simulink model "torqueBalancingR2015a"  (Simulink 8.5)
settings: Solver=FixedStepDiscrete  StartTime=0.0  StopTime="CONFIG.SIMULATION_TIME "  FixedStep=CONFIG.Ts  RelTol=1e-3
InitFcn:
  | cd(fileparts(which(bdroot)));
  | initTorqueBalancing;
values from neighbouring files (symbols this model uses):
  WBT_robotName = 'iCub'    [initTorqueBalancing.m]
undefined symbols (not defined in the file or in its folder): bVectorConstraints, CONFIG, ConstraintsMatrix, DiscIntNeverNeededParam, gain, references, reg, ROBOT_DOF, ROBOT_DOF_FOR_SIMULINK, sat, SM, sm
libraries: WBToolboxLibrary x141, simulink x6
(part 3 of 4)

== system torqueBalancingR2015a/State Machine/State machine Yoga and Coordinator/State Machine Yoga/visualise inertial/w_H_root_link1 ==
  qj : Inport
  inertial : Inport  Port=2
  "CoM6D ->  CoMXYZ1" : Selector  NumberOfDimensions=2  InputPortWidth=7  IndexOptions=Index vector (dialog),Index vector (dialog)  Indices=[1 2 3],[1 2 3]  OutputSizes=1,1
  Constant2 : Constant  Value=eye(4)
  Constant5 : Constant  Value=eye(4)
  Constant6 : Constant  Value=eye(4)
  Inv\* : Product  Inputs=/*  Multiplication=Matrix(*)
  Inv\*1 : Product  Inputs=/*  Multiplication=Matrix(*)
  Inv\*2 : Product  Inputs=/  Multiplication=Matrix(*)
  Product : Product  Multiplication=Matrix(*)
  Selector : Selector  InputPortWidth=12  IndexOptions=Index vector (dialog)  Indices=[4 5 6 ]  OutputSizes=1
  Subsystem : Subsystem
  Switch6 : Switch  Criteria=u2 > Threshold
  USE_IMU4EST_BASE : Constant  Value=CONFIG.USE_IMU4EST_BASE
  fromImuToHomogeousTransformFCN : MATLAB Function  TreatAsAtomicUnit=on
      settings: PermitHierarchicalResolution=ParametersOnly
  holder 1 : WBToolboxLibrary/Utilities/holder 
  holder 2 : WBToolboxLibrary/Utilities/holder 
  imu : WBToolboxLibrary/wholeBodyModel/Kinematics/Forward Kinematics  frameName='imu_frame'  robotName=WBT_robotName  localName=WBT_modelName  wbiFile=WBT_wbiFilename  wbiList=WBT_wbiList
  l_sole_acc : Scope
      settings: TimeRange=auto  LimitDataPoints=on  MaxDataPoints=5000  SaveToWorkspace=off  SaveName=ScopeData  YMin=-10  YMax=10  SampleTime=-1  DataFormat=Array
  link : WBToolboxLibrary/wholeBodyModel/Kinematics/Forward Kinematics  frameName=link_name  robotName=WBT_robotName  localName=WBT_modelName  wbiFile=WBT_wbiFilename  wbiList=WBT_wbiList
  root_link : WBToolboxLibrary/wholeBodyModel/Kinematics/Forward Kinematics  frameName='root_link'  robotName=WBT_robotName  localName=WBT_modelName  wbiFile=WBT_wbiFilename  wbiList=WBT_wbiList
  w_H_root : Outport
  wires:
  Constant5/1 -> imu/1
  Inv\*/1 -> holder 1/1, fromImuToHomogeousTransformFCN/1(imu_H_link), Inv\*2/1  "imu_H_link"
  imu/1 -> Inv\*/1
  Constant6/1 -> link/1
  Inv\*1/1 -> Switch6/3, fromImuToHomogeousTransformFCN/3(link_H_root)  "link_H_root"
  link/1 -> Inv\*1/1, Inv\*/2
  inertial/1 -> Selector/1, holder 2/1, fromImuToHomogeousTransformFCN/5(inertial)
  Switch6/1 -> w_H_root/1
  USE_IMU4EST_BASE/1 -> Switch6/2
  fromImuToHomogeousTransformFCN/1(w_H_root) -> Switch6/1
  Constant2/1 -> root_link/1
  qj/1 -> root_link/2, link/2, imu/2
  root_link/1 -> Inv\*1/2
  holder 1/1 -> fromImuToHomogeousTransformFCN/2(imu_H_link_0)
  holder 2/1 -> fromImuToHomogeousTransformFCN/4(inertial_0)
  Inv\*2/1 -> "CoM6D ->  CoMXYZ1"/1
  "CoM6D ->  CoMXYZ1"/1 -> Product/1  "l_sole_R_imu"
  Selector/1 -> Product/2  "imu_acce"
  Product/1 -> l_sole_acc/1
  Subsystem/1(Neck Position) -> fromImuToHomogeousTransformFCN/6(neck)

== system torqueBalancingR2015a/State Machine/State machine Yoga and Coordinator/State Machine Yoga/visualise inertial/w_H_root_link2 ==
  qj : Inport
  inertial : Inport  Port=2
  "CoM6D ->  CoMXYZ1" : Selector  NumberOfDimensions=2  InputPortWidth=7  IndexOptions=Index vector (dialog),Index vector (dialog)  Indices=[1 2 3],[1 2 3]  OutputSizes=1,1
  Constant2 : Constant  Value=eye(4)
  Constant5 : Constant  Value=eye(4)
  Constant6 : Constant  Value=eye(4)
  Inv\* : Product  Inputs=/*  Multiplication=Matrix(*)
  Inv\*1 : Product  Inputs=/*  Multiplication=Matrix(*)
  Inv\*2 : Product  Inputs=/  Multiplication=Matrix(*)
  Product : Product  Multiplication=Matrix(*)
  Selector : Selector  InputPortWidth=12  IndexOptions=Index vector (dialog)  Indices=[4 5 6 ]  OutputSizes=1
  Subsystem : Subsystem
  Switch6 : Switch  Criteria=u2 > Threshold
  USE_IMU4EST_BASE : Constant  Value=CONFIG.USE_IMU4EST_BASE
  fromImuToHomogeousTransformFCN : MATLAB Function  TreatAsAtomicUnit=on
      settings: PermitHierarchicalResolution=ParametersOnly
  holder 1 : WBToolboxLibrary/Utilities/holder 
  holder 2 : WBToolboxLibrary/Utilities/holder 
  imu : WBToolboxLibrary/wholeBodyModel/Kinematics/Forward Kinematics  frameName='imu_frame'  robotName=WBT_robotName  localName=WBT_modelName  wbiFile=WBT_wbiFilename  wbiList=WBT_wbiList
  l_sole_acc : Scope
      settings: TimeRange=auto  LimitDataPoints=on  MaxDataPoints=5000  SaveToWorkspace=off  SaveName=ScopeData  YMin=-10  YMax=10  SampleTime=-1  DataFormat=Array
  link : WBToolboxLibrary/wholeBodyModel/Kinematics/Forward Kinematics  frameName=link_name  robotName=WBT_robotName  localName=WBT_modelName  wbiFile=WBT_wbiFilename  wbiList=WBT_wbiList
  root_link : WBToolboxLibrary/wholeBodyModel/Kinematics/Forward Kinematics  frameName='root_link'  robotName=WBT_robotName  localName=WBT_modelName  wbiFile=WBT_wbiFilename  wbiList=WBT_wbiList
  w_H_root : Outport
  wires:
  Constant5/1 -> imu/1
  Inv\*/1 -> holder 1/1, fromImuToHomogeousTransformFCN/1(imu_H_link), Inv\*2/1  "imu_H_link"
  imu/1 -> Inv\*/1
  Constant6/1 -> link/1
  Inv\*1/1 -> Switch6/3, fromImuToHomogeousTransformFCN/3(link_H_root)  "link_H_root"
  link/1 -> Inv\*1/1, Inv\*/2
  inertial/1 -> Selector/1, holder 2/1, fromImuToHomogeousTransformFCN/5(inertial)
  Switch6/1 -> w_H_root/1
  USE_IMU4EST_BASE/1 -> Switch6/2
  fromImuToHomogeousTransformFCN/1(w_H_root) -> Switch6/1
  Constant2/1 -> root_link/1
  qj/1 -> root_link/2, link/2, imu/2
  root_link/1 -> Inv\*1/2
  holder 1/1 -> fromImuToHomogeousTransformFCN/2(imu_H_link_0)
  holder 2/1 -> fromImuToHomogeousTransformFCN/4(inertial_0)
  Inv\*2/1 -> "CoM6D ->  CoMXYZ1"/1
  "CoM6D ->  CoMXYZ1"/1 -> Product/1  "l_sole_R_imu"
  Selector/1 -> Product/2  "imu_acce"
  Product/1 -> l_sole_acc/1
  Subsystem/1(Neck Position) -> fromImuToHomogeousTransformFCN/6(neck)

== system torqueBalancingR2015a/State Machine/State machine Yoga and Coordinator/State Machine Yoga/w_H_root_link1/Subsystem ==
  Constant : Constant  Value=zeros(3,1)
  Gain : Gain  Gain=pi/180
  Head state : WBToolboxLibrary/Utilities/Yarp Read  portName=['/',WBT_robotName, '/head/state:o']  signalSize=6  blocking=off  timestamp=off  autoconnect=on  errorOnConnection=off
  Selector1 : Selector  InputPortWidth=6  IndexOptions=Index vector (dialog)  Indices=[1:3]  OutputSizes=1
  Switch : Switch  Criteria=u2 > Threshold
  USE_IMU4EST_BASE1 : Constant  Value=CONFIG.CORRECT_NECK_IMU
  Neck Position : Outport
  wires:
  Head state/1 -> Gain/1
  Selector1/1 -> Switch/1  "neck"
  USE_IMU4EST_BASE1/1 -> Switch/2
  Switch/1 -> Neck Position/1
  Gain/1 -> Selector1/1
  Constant/1 -> Switch/3

== system torqueBalancingR2015a/State Machine/State machine Yoga and Coordinator/State Machine Yoga/w_H_root_link2/Subsystem ==
  Constant : Constant  Value=zeros(3,1)
  Gain : Gain  Gain=pi/180
  Head state : WBToolboxLibrary/Utilities/Yarp Read  portName=['/',WBT_robotName, '/head/state:o']  signalSize=6  blocking=off  timestamp=off  autoconnect=on  errorOnConnection=off
  Selector1 : Selector  InputPortWidth=6  IndexOptions=Index vector (dialog)  Indices=[1:3]  OutputSizes=1
  Switch : Switch  Criteria=u2 > Threshold
  USE_IMU4EST_BASE1 : Constant  Value=CONFIG.CORRECT_NECK_IMU
  Neck Position : Outport
  wires:
  Head state/1 -> Gain/1
  Selector1/1 -> Switch/1  "neck"
  USE_IMU4EST_BASE1/1 -> Switch/2
  Switch/1 -> Neck Position/1
  Gain/1 -> Selector1/1
  Constant/1 -> Switch/3

== system torqueBalancingR2015a/State Machine/State machine walking/State Machine Walking/Compute w_H_b transform/w_H_root_link1 ==
  qj : Inport
  inertial : Inport  Port=2
  "CoM6D ->  CoMXYZ1" : Selector  NumberOfDimensions=2  InputPortWidth=7  IndexOptions=Index vector (dialog),Index vector (dialog)  Indices=[1 2 3],[1 2 3]  OutputSizes=1,1
  Constant2 : Constant  Value=eye(4)
  Constant5 : Constant  Value=eye(4)
  Constant6 : Constant  Value=eye(4)
  Inv\* : Product  Inputs=/*  Multiplication=Matrix(*)
  Inv\*1 : Product  Inputs=/*  Multiplication=Matrix(*)
  Inv\*2 : Product  Inputs=/  Multiplication=Matrix(*)
  Product : Product  Multiplication=Matrix(*)
  Selector : Selector  InputPortWidth=12  IndexOptions=Index vector (dialog)  Indices=[4 5 6 ]  OutputSizes=1
  Subsystem : Subsystem
  Switch6 : Switch  Criteria=u2 > Threshold
  USE_IMU4EST_BASE : Constant  Value=CONFIG.USE_IMU4EST_BASE
  fromImuToHomogeousTransformFCN : MATLAB Function  TreatAsAtomicUnit=on
      settings: PermitHierarchicalResolution=ParametersOnly
  holder 1 : WBToolboxLibrary/Utilities/holder 
  holder 2 : WBToolboxLibrary/Utilities/holder 
  imu : WBToolboxLibrary/wholeBodyModel/Kinematics/Forward Kinematics  frameName='imu_frame'  robotName=WBT_robotName  localName=WBT_modelName  wbiFile=WBT_wbiFilename  wbiList=WBT_wbiList
  l_sole_acc : Scope
      settings: TimeRange=auto  LimitDataPoints=on  MaxDataPoints=5000  SaveToWorkspace=off  SaveName=ScopeData  YMin=-10  YMax=10  SampleTime=-1  DataFormat=Array
  link : WBToolboxLibrary/wholeBodyModel/Kinematics/Forward Kinematics  frameName=link_name  robotName=WBT_robotName  localName=WBT_modelName  wbiFile=WBT_wbiFilename  wbiList=WBT_wbiList
  root_link : WBToolboxLibrary/wholeBodyModel/Kinematics/Forward Kinematics  frameName='root_link'  robotName=WBT_robotName  localName=WBT_modelName  wbiFile=WBT_wbiFilename  wbiList=WBT_wbiList
  w_H_root : Outport
  wires:
  Constant5/1 -> imu/1
  Inv\*/1 -> holder 1/1, fromImuToHomogeousTransformFCN/1(imu_H_link), Inv\*2/1  "imu_H_link"
  imu/1 -> Inv\*/1
  Constant6/1 -> link/1
  Inv\*1/1 -> Switch6/3, fromImuToHomogeousTransformFCN/3(link_H_root)  "link_H_root"
  link/1 -> Inv\*1/1, Inv\*/2
  inertial/1 -> Selector/1, holder 2/1, fromImuToHomogeousTransformFCN/5(inertial)
  Switch6/1 -> w_H_root/1
  USE_IMU4EST_BASE/1 -> Switch6/2
  fromImuToHomogeousTransformFCN/1(w_H_root) -> Switch6/1
  Constant2/1 -> root_link/1
  qj/1 -> root_link/2, link/2, imu/2
  root_link/1 -> Inv\*1/2
  holder 1/1 -> fromImuToHomogeousTransformFCN/2(imu_H_link_0)
  holder 2/1 -> fromImuToHomogeousTransformFCN/4(inertial_0)
  Inv\*2/1 -> "CoM6D ->  CoMXYZ1"/1
  "CoM6D ->  CoMXYZ1"/1 -> Product/1  "l_sole_R_imu"
  Selector/1 -> Product/2  "imu_acce"
  Product/1 -> l_sole_acc/1
  Subsystem/1(Neck Position) -> fromImuToHomogeousTransformFCN/6(neck)

== system torqueBalancingR2015a/State Machine/State machine walking/State Machine Walking/Compute w_H_b transform/w_H_root_link2 ==
  qj : Inport
  inertial : Inport  Port=2
  "CoM6D ->  CoMXYZ1" : Selector  NumberOfDimensions=2  InputPortWidth=7  IndexOptions=Index vector (dialog),Index vector (dialog)  Indices=[1 2 3],[1 2 3]  OutputSizes=1,1
  Constant2 : Constant  Value=eye(4)
  Constant5 : Constant  Value=eye(4)
  Constant6 : Constant  Value=eye(4)
  Inv\* : Product  Inputs=/*  Multiplication=Matrix(*)
  Inv\*1 : Product  Inputs=/*  Multiplication=Matrix(*)
  Inv\*2 : Product  Inputs=/  Multiplication=Matrix(*)
  Product : Product  Multiplication=Matrix(*)
  Selector : Selector  InputPortWidth=12  IndexOptions=Index vector (dialog)  Indices=[4 5 6 ]  OutputSizes=1
  Subsystem : Subsystem
  Switch6 : Switch  Criteria=u2 > Threshold
  USE_IMU4EST_BASE : Constant  Value=CONFIG.USE_IMU4EST_BASE
  fromImuToHomogeousTransformFCN : MATLAB Function  TreatAsAtomicUnit=on
      settings: PermitHierarchicalResolution=ParametersOnly
  holder 1 : WBToolboxLibrary/Utilities/holder 
  holder 2 : WBToolboxLibrary/Utilities/holder 
  imu : WBToolboxLibrary/wholeBodyModel/Kinematics/Forward Kinematics  frameName='imu_frame'  robotName=WBT_robotName  localName=WBT_modelName  wbiFile=WBT_wbiFilename  wbiList=WBT_wbiList
  l_sole_acc : Scope
      settings: TimeRange=auto  LimitDataPoints=on  MaxDataPoints=5000  SaveToWorkspace=off  SaveName=ScopeData  YMin=-10  YMax=10  SampleTime=-1  DataFormat=Array
  link : WBToolboxLibrary/wholeBodyModel/Kinematics/Forward Kinematics  frameName=link_name  robotName=WBT_robotName  localName=WBT_modelName  wbiFile=WBT_wbiFilename  wbiList=WBT_wbiList
  root_link : WBToolboxLibrary/wholeBodyModel/Kinematics/Forward Kinematics  frameName='root_link'  robotName=WBT_robotName  localName=WBT_modelName  wbiFile=WBT_wbiFilename  wbiList=WBT_wbiList
  w_H_root : Outport
  wires:
  Constant5/1 -> imu/1
  Inv\*/1 -> holder 1/1, fromImuToHomogeousTransformFCN/1(imu_H_link), Inv\*2/1  "imu_H_link"
  imu/1 -> Inv\*/1
  Constant6/1 -> link/1
  Inv\*1/1 -> Switch6/3, fromImuToHomogeousTransformFCN/3(link_H_root)  "link_H_root"
  link/1 -> Inv\*1/1, Inv\*/2
  inertial/1 -> Selector/1, holder 2/1, fromImuToHomogeousTransformFCN/5(inertial)
  Switch6/1 -> w_H_root/1
  USE_IMU4EST_BASE/1 -> Switch6/2
  fromImuToHomogeousTransformFCN/1(w_H_root) -> Switch6/1
  Constant2/1 -> root_link/1
  qj/1 -> root_link/2, link/2, imu/2
  root_link/1 -> Inv\*1/2
  holder 1/1 -> fromImuToHomogeousTransformFCN/2(imu_H_link_0)
  holder 2/1 -> fromImuToHomogeousTransformFCN/4(inertial_0)
  Inv\*2/1 -> "CoM6D ->  CoMXYZ1"/1
  "CoM6D ->  CoMXYZ1"/1 -> Product/1  "l_sole_R_imu"
  Selector/1 -> Product/2  "imu_acce"
  Product/1 -> l_sole_acc/1
  Subsystem/1(Neck Position) -> fromImuToHomogeousTransformFCN/6(neck)

== system torqueBalancingR2015a/State Machine/State machine walking/State Machine Walking/visualise inertial/Visualize hom transf1 ==
  H : Inport
  "CoM6D ->  CoMXYZ1" : Selector  NumberOfDimensions=2  InputPortWidth=7  IndexOptions=Index vector (dialog),Index vector (dialog)  Indices=[1 2 3],[1 2 3]  OutputSizes=1,1
  "CoM6D ->  CoMXYZ2" : Selector  NumberOfDimensions=2  InputPortWidth=7  IndexOptions=Index vector (dialog),Index vector (dialog)  Indices=[1 2 3],[4]  OutputSizes=1,1
  Hom : Scope
      settings: TimeRange=auto  LimitDataPoints=on  MaxDataPoints=5000  SaveToWorkspace=off  SaveName=ScopeData  YMin=-10  YMax=10  SampleTime=-1  DataFormat=Array
  R : Scope
      settings: TimeRange=auto  LimitDataPoints=on  MaxDataPoints=5000  SaveToWorkspace=off  SaveName=ScopeData  YMin=-10  YMax=10  SampleTime=-1  DataFormat=Array
  p : Scope
      settings: TimeRange=auto  LimitDataPoints=on  MaxDataPoints=5000  SaveToWorkspace=off  SaveName=ScopeData  YMin=-10  YMax=10  SampleTime=-1  DataFormat=Array
  wires:
  "CoM6D ->  CoMXYZ1"/1 -> R/1
  "CoM6D ->  CoMXYZ2"/1 -> p/1
  H/1 -> "CoM6D ->  CoMXYZ2"/1, Hom/1, "CoM6D ->  CoMXYZ1"/1

== system torqueBalancingR2015a/State Machine/State machine walking/State Machine Walking/visualise inertial/Visualize hom transf2 ==
  H : Inport
  "CoM6D ->  CoMXYZ1" : Selector  NumberOfDimensions=2  InputPortWidth=7  IndexOptions=Index vector (dialog),Index vector (dialog)  Indices=[1 2 3],[1 2 3]  OutputSizes=1,1
  "CoM6D ->  CoMXYZ2" : Selector  NumberOfDimensions=2  InputPortWidth=7  IndexOptions=Index vector (dialog),Index vector (dialog)  Indices=[1 2 3],[4]  OutputSizes=1,1
  Hom : Scope
      settings: TimeRange=auto  LimitDataPoints=on  MaxDataPoints=5000  SaveToWorkspace=off  SaveName=ScopeData  YMin=-10  YMax=10  SampleTime=-1  DataFormat=Array
  R : Scope
      settings: TimeRange=auto  LimitDataPoints=on  MaxDataPoints=5000  SaveToWorkspace=off  SaveName=ScopeData  YMin=-10  YMax=10  SampleTime=-1  DataFormat=Array
  p : Scope
      settings: TimeRange=auto  LimitDataPoints=on  MaxDataPoints=5000  SaveToWorkspace=off  SaveName=ScopeData  YMin=-10  YMax=10  SampleTime=-1  DataFormat=Array
  wires:
  "CoM6D ->  CoMXYZ1"/1 -> R/1
  "CoM6D ->  CoMXYZ2"/1 -> p/1
  H/1 -> "CoM6D ->  CoMXYZ2"/1, Hom/1, "CoM6D ->  CoMXYZ1"/1

== system torqueBalancingR2015a/State Machine/State machine walking/State Machine Walking/visualise inertial/Visualize hom transf3 ==
  H : Inport
  "CoM6D ->  CoMXYZ1" : Selector  NumberOfDimensions=2  InputPortWidth=7  IndexOptions=Index vector (dialog),Index vector (dialog)  Indices=[1 2 3],[1 2 3]  OutputSizes=1,1
  "CoM6D ->  CoMXYZ2" : Selector  NumberOfDimensions=2  InputPortWidth=7  IndexOptions=Index vector (dialog),Index vector (dialog)  Indices=[1 2 3],[4]  OutputSizes=1,1
  Hom : Scope
      settings: TimeRange=auto  LimitDataPoints=on  MaxDataPoints=5000  SaveToWorkspace=off  SaveName=ScopeData  YMin=-10  YMax=10  SampleTime=-1  DataFormat=Array
  R : Scope
      settings: TimeRange=auto  LimitDataPoints=on  MaxDataPoints=5000  SaveToWorkspace=off  SaveName=ScopeData  YMin=-10  YMax=10  SampleTime=-1  DataFormat=Array
  p : Scope
      settings: TimeRange=auto  LimitDataPoints=on  MaxDataPoints=5000  SaveToWorkspace=off  SaveName=ScopeData  YMin=-10  YMax=10  SampleTime=-1  DataFormat=Array
  wires:
  "CoM6D ->  CoMXYZ1"/1 -> R/1
  "CoM6D ->  CoMXYZ2"/1 -> p/1
  H/1 -> "CoM6D ->  CoMXYZ2"/1, Hom/1, "CoM6D ->  CoMXYZ1"/1

== system torqueBalancingR2015a/State Machine/State machine walking/State Machine Walking/visualise inertial/Visualize hom transf4 ==
  H : Inport
  "CoM6D ->  CoMXYZ1" : Selector  NumberOfDimensions=2  InputPortWidth=7  IndexOptions=Index vector (dialog),Index vector (dialog)  Indices=[1 2 3],[1 2 3]  OutputSizes=1,1
  "CoM6D ->  CoMXYZ2" : Selector  NumberOfDimensions=2  InputPortWidth=7  IndexOptions=Index vector (dialog),Index vector (dialog)  Indices=[1 2 3],[4]  OutputSizes=1,1
  Hom : Scope
      settings: TimeRange=auto  LimitDataPoints=on  MaxDataPoints=5000  SaveToWorkspace=off  SaveName=ScopeData  YMin=-10  YMax=10  SampleTime=-1  DataFormat=Array
  R : Scope
      settings: TimeRange=auto  LimitDataPoints=on  MaxDataPoints=5000  SaveToWorkspace=off  SaveName=ScopeData  YMin=-10  YMax=10  SampleTime=-1  DataFormat=Array
  p : Scope
      settings: TimeRange=auto  LimitDataPoints=on  MaxDataPoints=5000  SaveToWorkspace=off  SaveName=ScopeData  YMin=-10  YMax=10  SampleTime=-1  DataFormat=Array
  wires:
  "CoM6D ->  CoMXYZ1"/1 -> R/1
  "CoM6D ->  CoMXYZ2"/1 -> p/1
  H/1 -> "CoM6D ->  CoMXYZ2"/1, Hom/1, "CoM6D ->  CoMXYZ1"/1

== system torqueBalancingR2015a/State Machine/State machine walking/State Machine Walking/visualise inertial/Visualize hom transf5 ==
  H : Inport
  "CoM6D ->  CoMXYZ1" : Selector  NumberOfDimensions=2  InputPortWidth=7  IndexOptions=Index vector (dialog),Index vector (dialog)  Indices=[1 2 3],[1 2 3]  OutputSizes=1,1
  "CoM6D ->  CoMXYZ2" : Selector  NumberOfDimensions=2  InputPortWidth=7  IndexOptions=Index vector (dialog),Index vector (dialog)  Indices=[1 2 3],[4]  OutputSizes=1,1
  Hom : Scope
      settings: TimeRange=auto  LimitDataPoints=on  MaxDataPoints=5000  SaveToWorkspace=off  SaveName=ScopeData  YMin=-10  YMax=10  SampleTime=-1  DataFormat=Array
  R : Scope
      settings: TimeRange=auto  LimitDataPoints=on  MaxDataPoints=5000  SaveToWorkspace=off  SaveName=ScopeData  YMin=-10  YMax=10  SampleTime=-1  DataFormat=Array
  p : Scope
      settings: TimeRange=auto  LimitDataPoints=on  MaxDataPoints=5000  SaveToWorkspace=off  SaveName=ScopeData  YMin=-10  YMax=10  SampleTime=-1  DataFormat=Array
  wires:
  "CoM6D ->  CoMXYZ1"/1 -> R/1
  "CoM6D ->  CoMXYZ2"/1 -> p/1
  H/1 -> "CoM6D ->  CoMXYZ2"/1, Hom/1, "CoM6D ->  CoMXYZ1"/1

== system torqueBalancingR2015a/State Machine/State machine walking/State Machine Walking/visualise inertial/Visualize hom transf7 ==
  H : Inport
  "CoM6D ->  CoMXYZ1" : Selector  NumberOfDimensions=2  InputPortWidth=7  IndexOptions=Index vector (dialog),Index vector (dialog)  Indices=[1 2 3],[1 2 3]  OutputSizes=1,1
  "CoM6D ->  CoMXYZ2" : Selector  NumberOfDimensions=2  InputPortWidth=7  IndexOptions=Index vector (dialog),Index vector (dialog)  Indices=[1 2 3],[4]  OutputSizes=1,1
  Hom : Scope
      settings: TimeRange=auto  LimitDataPoints=on  MaxDataPoints=5000  SaveToWorkspace=off  SaveName=ScopeData  YMin=-10  YMax=10  SampleTime=-1  DataFormat=Array
  R : Scope
      settings: TimeRange=auto  LimitDataPoints=on  MaxDataPoints=5000  SaveToWorkspace=off  SaveName=ScopeData  YMin=-10  YMax=10  SampleTime=-1  DataFormat=Array
  p : Scope
      settings: TimeRange=auto  LimitDataPoints=on  MaxDataPoints=5000  SaveToWorkspace=off  SaveName=ScopeData  YMin=-10  YMax=10  SampleTime=-1  DataFormat=Array
  wires:
  "CoM6D ->  CoMXYZ1"/1 -> R/1
  "CoM6D ->  CoMXYZ2"/1 -> p/1
  H/1 -> "CoM6D ->  CoMXYZ2"/1, Hom/1, "CoM6D ->  CoMXYZ1"/1

== system torqueBalancingR2015a/State Machine/State machine walking/State Machine Walking/visualise inertial/l_sole_H_root_link1 ==
  qj : Inport
  Constant5 : Constant  Value=eye(4)
  Constant6 : Constant  Value=eye(4)
  Inv\* : Product  Inputs=/*  Multiplication=Matrix(*)
  Visualize hom transf7 : Subsystem
  link_name : WBToolboxLibrary/wholeBodyModel/Kinematics/Forward Kinematics  frameName=link_name  robotName=WBT_robotName  localName=WBT_modelName  wbiFile=WBT_wbiFilename  wbiList=WBT_wbiList
  root_link : WBToolboxLibrary/wholeBodyModel/Kinematics/Forward Kinematics  frameName=FRAMES.BASE  robotName=WBT_robotName  localName=WBT_modelName  wbiFile=WBT_wbiFilename  wbiList=WBT_wbiList
  link_name_H_root_link : Outport
  wires:
  Constant5/1 -> link_name/1
  Inv\*/1 -> link_name_H_root_link/1  "link_name_H_root_link"
  link_name/1 -> Inv\*/1
  Constant6/1 -> root_link/1
  qj/1 -> root_link/2, link_name/2
  root_link/1 -> Visualize hom transf7/1(H), Inv\*/2

== system torqueBalancingR2015a/State Machine/State machine walking/State Machine Walking/visualise inertial/l_sole_H_root_link2 ==
  qj : Inport
  Constant5 : Constant  Value=eye(4)
  Constant6 : Constant  Value=eye(4)
  Inv\* : Product  Inputs=/*  Multiplication=Matrix(*)
  Visualize hom transf7 : Subsystem
  link_name : WBToolboxLibrary/wholeBodyModel/Kinematics/Forward Kinematics  frameName=link_name  robotName=WBT_robotName  localName=WBT_modelName  wbiFile=WBT_wbiFilename  wbiList=WBT_wbiList
  root_link : WBToolboxLibrary/wholeBodyModel/Kinematics/Forward Kinematics  frameName=FRAMES.BASE  robotName=WBT_robotName  localName=WBT_modelName  wbiFile=WBT_wbiFilename  wbiList=WBT_wbiList
  link_name_H_root_link : Outport
  wires:
  Constant5/1 -> link_name/1
  Inv\*/1 -> link_name_H_root_link/1  "link_name_H_root_link"
  link_name/1 -> Inv\*/1
  Constant6/1 -> root_link/1
  qj/1 -> root_link/2, link_name/2
  root_link/1 -> Visualize hom transf7/1(H), Inv\*/2

== system torqueBalancingR2015a/State Machine/State machine walking/State Machine Walking/visualise inertial/w_H_root_link1 ==
  qj : Inport
  inertial : Inport  Port=2
  "CoM6D ->  CoMXYZ1" : Selector  NumberOfDimensions=2  InputPortWidth=7  IndexOptions=Index vector (dialog),Index vector (dialog)  Indices=[1 2 3],[1 2 3]  OutputSizes=1,1
  Constant2 : Constant  Value=eye(4)
  Constant5 : Constant  Value=eye(4)
  Constant6 : Constant  Value=eye(4)
  Inv\* : Product  Inputs=/*  Multiplication=Matrix(*)
  Inv\*1 : Product  Inputs=/*  Multiplication=Matrix(*)
  Inv\*2 : Product  Inputs=/  Multiplication=Matrix(*)
  Product : Product  Multiplication=Matrix(*)
  Selector : Selector  InputPortWidth=12  IndexOptions=Index vector (dialog)  Indices=[4 5 6 ]  OutputSizes=1
  Subsystem : Subsystem
  Switch6 : Switch  Criteria=u2 > Threshold
  USE_IMU4EST_BASE : Constant  Value=CONFIG.USE_IMU4EST_BASE
  fromImuToHomogeousTransformFCN : MATLAB Function  TreatAsAtomicUnit=on
      settings: PermitHierarchicalResolution=ParametersOnly
  holder 1 : WBToolboxLibrary/Utilities/holder 
  holder 2 : WBToolboxLibrary/Utilities/holder 
  imu : WBToolboxLibrary/wholeBodyModel/Kinematics/Forward Kinematics  frameName='imu_frame'  robotName=WBT_robotName  localName=WBT_modelName  wbiFile=WBT_wbiFilename  wbiList=WBT_wbiList
  l_sole_acc : Scope
      settings: TimeRange=auto  LimitDataPoints=on  MaxDataPoints=5000  SaveToWorkspace=off  SaveName=ScopeData  YMin=-10  YMax=10  SampleTime=-1  DataFormat=Array
  link : WBToolboxLibrary/wholeBodyModel/Kinematics/Forward Kinematics  frameName=link_name  robotName=WBT_robotName  localName=WBT_modelName  wbiFile=WBT_wbiFilename  wbiList=WBT_wbiList
  root_link : WBToolboxLibrary/wholeBodyModel/Kinematics/Forward Kinematics  frameName='root_link'  robotName=WBT_robotName  localName=WBT_modelName  wbiFile=WBT_wbiFilename  wbiList=WBT_wbiList
  w_H_root : Outport
  wires:
  Constant5/1 -> imu/1
  Inv\*/1 -> holder 1/1, fromImuToHomogeousTransformFCN/1(imu_H_link), Inv\*2/1  "imu_H_link"
  imu/1 -> Inv\*/1
  Constant6/1 -> link/1
  Inv\*1/1 -> Switch6/3, fromImuToHomogeousTransformFCN/3(link_H_root)  "link_H_root"
  link/1 -> Inv\*1/1, Inv\*/2
  inertial/1 -> Selector/1, holder 2/1, fromImuToHomogeousTransformFCN/5(inertial)
  Switch6/1 -> w_H_root/1
  USE_IMU4EST_BASE/1 -> Switch6/2
  fromImuToHomogeousTransformFCN/1(w_H_root) -> Switch6/1
  Constant2/1 -> root_link/1
  qj/1 -> root_link/2, link/2, imu/2
  root_link/1 -> Inv\*1/2
  holder 1/1 -> fromImuToHomogeousTransformFCN/2(imu_H_link_0)
  holder 2/1 -> fromImuToHomogeousTransformFCN/4(inertial_0)
  Inv\*2/1 -> "CoM6D ->  CoMXYZ1"/1
  "CoM6D ->  CoMXYZ1"/1 -> Product/1  "l_sole_R_imu"
  Selector/1 -> Product/2  "imu_acce"
  Product/1 -> l_sole_acc/1
  Subsystem/1(Neck Position) -> fromImuToHomogeousTransformFCN/6(neck)

== system torqueBalancingR2015a/State Machine/State machine walking/State Machine Walking/visualise inertial/w_H_root_link2 ==
  qj : Inport
  inertial : Inport  Port=2
  "CoM6D ->  CoMXYZ1" : Selector  NumberOfDimensions=2  InputPortWidth=7  IndexOptions=Index vector (dialog),Index vector (dialog)  Indices=[1 2 3],[1 2 3]  OutputSizes=1,1
  Constant2 : Constant  Value=eye(4)
  Constant5 : Constant  Value=eye(4)
  Constant6 : Constant  Value=eye(4)
  Inv\* : Product  Inputs=/*  Multiplication=Matrix(*)
  Inv\*1 : Product  Inputs=/*  Multiplication=Matrix(*)
  Inv\*2 : Product  Inputs=/  Multiplication=Matrix(*)
  Product : Product  Multiplication=Matrix(*)
  Selector : Selector  InputPortWidth=12  IndexOptions=Index vector (dialog)  Indices=[4 5 6 ]  OutputSizes=1
  Subsystem : Subsystem
  Switch6 : Switch  Criteria=u2 > Threshold
  USE_IMU4EST_BASE : Constant  Value=CONFIG.USE_IMU4EST_BASE
  fromImuToHomogeousTransformFCN : MATLAB Function  TreatAsAtomicUnit=on
      settings: PermitHierarchicalResolution=ParametersOnly
  holder 1 : WBToolboxLibrary/Utilities/holder 
  holder 2 : WBToolboxLibrary/Utilities/holder 
  imu : WBToolboxLibrary/wholeBodyModel/Kinematics/Forward Kinematics  frameName='imu_frame'  robotName=WBT_robotName  localName=WBT_modelName  wbiFile=WBT_wbiFilename  wbiList=WBT_wbiList
  l_sole_acc : Scope
      settings: TimeRange=auto  LimitDataPoints=on  MaxDataPoints=5000  SaveToWorkspace=off  SaveName=ScopeData  YMin=-10  YMax=10  SampleTime=-1  DataFormat=Array
  link : WBToolboxLibrary/wholeBodyModel/Kinematics/Forward Kinematics  frameName=link_name  robotName=WBT_robotName  localName=WBT_modelName  wbiFile=WBT_wbiFilename  wbiList=WBT_wbiList
  root_link : WBToolboxLibrary/wholeBodyModel/Kinematics/Forward Kinematics  frameName='root_link'  robotName=WBT_robotName  localName=WBT_modelName  wbiFile=WBT_wbiFilename  wbiList=WBT_wbiList
  w_H_root : Outport
  wires:
  Constant5/1 -> imu/1
  Inv\*/1 -> holder 1/1, fromImuToHomogeousTransformFCN/1(imu_H_link), Inv\*2/1  "imu_H_link"
  imu/1 -> Inv\*/1
  Constant6/1 -> link/1
  Inv\*1/1 -> Switch6/3, fromImuToHomogeousTransformFCN/3(link_H_root)  "link_H_root"
  link/1 -> Inv\*1/1, Inv\*/2
  inertial/1 -> Selector/1, holder 2/1, fromImuToHomogeousTransformFCN/5(inertial)
  Switch6/1 -> w_H_root/1
  USE_IMU4EST_BASE/1 -> Switch6/2
  fromImuToHomogeousTransformFCN/1(w_H_root) -> Switch6/1
  Constant2/1 -> root_link/1
  qj/1 -> root_link/2, link/2, imu/2
  root_link/1 -> Inv\*1/2
  holder 1/1 -> fromImuToHomogeousTransformFCN/2(imu_H_link_0)
  holder 2/1 -> fromImuToHomogeousTransformFCN/4(inertial_0)
  Inv\*2/1 -> "CoM6D ->  CoMXYZ1"/1
  "CoM6D ->  CoMXYZ1"/1 -> Product/1  "l_sole_R_imu"
  Selector/1 -> Product/2  "imu_acce"
  Product/1 -> l_sole_acc/1
  Subsystem/1(Neck Position) -> fromImuToHomogeousTransformFCN/6(neck)

== system torqueBalancingR2015a/State Machine/State machine Yoga and Coordinator/State Machine Yoga/visualise inertial/l_sole_H_root_link1/Visualize hom transf7 ==
  H : Inport
  "CoM6D ->  CoMXYZ1" : Selector  NumberOfDimensions=2  InputPortWidth=7  IndexOptions=Index vector (dialog),Index vector (dialog)  Indices=[1 2 3],[1 2 3]  OutputSizes=1,1
  "CoM6D ->  CoMXYZ2" : Selector  NumberOfDimensions=2  InputPortWidth=7  IndexOptions=Index vector (dialog),Index vector (dialog)  Indices=[1 2 3],[4]  OutputSizes=1,1
  Hom : Scope
      settings: TimeRange=auto  LimitDataPoints=on  MaxDataPoints=5000  SaveToWorkspace=off  SaveName=ScopeData  YMin=-10  YMax=10  SampleTime=-1  DataFormat=Array
  R : Scope
      settings: TimeRange=auto  LimitDataPoints=on  MaxDataPoints=5000  SaveToWorkspace=off  SaveName=ScopeData  YMin=-10  YMax=10  SampleTime=-1  DataFormat=Array
  p : Scope
      settings: TimeRange=auto  LimitDataPoints=on  MaxDataPoints=5000  SaveToWorkspace=off  SaveName=ScopeData  YMin=-10  YMax=10  SampleTime=-1  DataFormat=Array
  wires:
  "CoM6D ->  CoMXYZ1"/1 -> R/1
  "CoM6D ->  CoMXYZ2"/1 -> p/1
  H/1 -> "CoM6D ->  CoMXYZ2"/1, Hom/1, "CoM6D ->  CoMXYZ1"/1

== system torqueBalancingR2015a/State Machine/State machine Yoga and Coordinator/State Machine Yoga/visualise inertial/l_sole_H_root_link2/Visualize hom transf7 ==
  H : Inport
  "CoM6D ->  CoMXYZ1" : Selector  NumberOfDimensions=2  InputPortWidth=7  IndexOptions=Index vector (dialog),Index vector (dialog)  Indices=[1 2 3],[1 2 3]  OutputSizes=1,1
  "CoM6D ->  CoMXYZ2" : Selector  NumberOfDimensions=2  InputPortWidth=7  IndexOptions=Index vector (dialog),Index vector (dialog)  Indices=[1 2 3],[4]  OutputSizes=1,1
  Hom : Scope
      settings: TimeRange=auto  LimitDataPoints=on  MaxDataPoints=5000  SaveToWorkspace=off  SaveName=ScopeData  YMin=-10  YMax=10  SampleTime=-1  DataFormat=Array
  R : Scope
      settings: TimeRange=auto  LimitDataPoints=on  MaxDataPoints=5000  SaveToWorkspace=off  SaveName=ScopeData  YMin=-10  YMax=10  SampleTime=-1  DataFormat=Array
  p : Scope
      settings: TimeRange=auto  LimitDataPoints=on  MaxDataPoints=5000  SaveToWorkspace=off  SaveName=ScopeData  YMin=-10  YMax=10  SampleTime=-1  DataFormat=Array
  wires:
  "CoM6D ->  CoMXYZ1"/1 -> R/1
  "CoM6D ->  CoMXYZ2"/1 -> p/1
  H/1 -> "CoM6D ->  CoMXYZ2"/1, Hom/1, "CoM6D ->  CoMXYZ1"/1

== system torqueBalancingR2015a/State Machine/State machine Yoga and Coordinator/State Machine Yoga/visualise inertial/w_H_root_link1/Subsystem ==
  Constant : Constant  Value=zeros(3,1)
  Gain : Gain  Gain=pi/180
  Head state : WBToolboxLibrary/Utilities/Yarp Read  portName=['/',WBT_robotName, '/head/state:o']  signalSize=6  blocking=off  timestamp=off  autoconnect=on  errorOnConnection=off
  Selector1 : Selector  InputPortWidth=6  IndexOptions=Index vector (dialog)  Indices=[1:3]  OutputSizes=1
  Switch : Switch  Criteria=u2 > Threshold
  USE_IMU4EST_BASE1 : Constant  Value=CONFIG.CORRECT_NECK_IMU
  Neck Position : Outport
  wires:
  Head state/1 -> Gain/1
  Selector1/1 -> Switch/1  "neck"
  USE_IMU4EST_BASE1/1 -> Switch/2
  Switch/1 -> Neck Position/1
  Gain/1 -> Selector1/1
  Constant/1 -> Switch/3

== system torqueBalancingR2015a/State Machine/State machine Yoga and Coordinator/State Machine Yoga/visualise inertial/w_H_root_link2/Subsystem ==
  Constant : Constant  Value=zeros(3,1)
  Gain : Gain  Gain=pi/180
  Head state : WBToolboxLibrary/Utilities/Yarp Read  portName=['/',WBT_robotName, '/head/state:o']  signalSize=6  blocking=off  timestamp=off  autoconnect=on  errorOnConnection=off
  Selector1 : Selector  InputPortWidth=6  IndexOptions=Index vector (dialog)  Indices=[1:3]  OutputSizes=1
  Switch : Switch  Criteria=u2 > Threshold
  USE_IMU4EST_BASE1 : Constant  Value=CONFIG.CORRECT_NECK_IMU
  Neck Position : Outport
  wires:
  Head state/1 -> Gain/1
  Selector1/1 -> Switch/1  "neck"
  USE_IMU4EST_BASE1/1 -> Switch/2
  Switch/1 -> Neck Position/1
  Gain/1 -> Selector1/1
  Constant/1 -> Switch/3

== system torqueBalancingR2015a/State Machine/State machine walking/State Machine Walking/Compute w_H_b transform/w_H_root_link1/Subsystem ==
  Constant : Constant  Value=zeros(3,1)
  Gain : Gain  Gain=pi/180
  Head state : WBToolboxLibrary/Utilities/Yarp Read  portName=['/',WBT_robotName, '/head/state:o']  signalSize=6  blocking=off  timestamp=off  autoconnect=on  errorOnConnection=off
  Selector1 : Selector  InputPortWidth=6  IndexOptions=Index vector (dialog)  Indices=[1:3]  OutputSizes=1
  Switch : Switch  Criteria=u2 > Threshold
  USE_IMU4EST_BASE1 : Constant  Value=CONFIG.CORRECT_NECK_IMU
  Neck Position : Outport
  wires:
  Head state/1 -> Gain/1
  Selector1/1 -> Switch/1  "neck"
  USE_IMU4EST_BASE1/1 -> Switch/2
  Switch/1 -> Neck Position/1
  Gain/1 -> Selector1/1
  Constant/1 -> Switch/3

== system torqueBalancingR2015a/State Machine/State machine walking/State Machine Walking/Compute w_H_b transform/w_H_root_link2/Subsystem ==
  Constant : Constant  Value=zeros(3,1)
  Gain : Gain  Gain=pi/180
  Head state : WBToolboxLibrary/Utilities/Yarp Read  portName=['/',WBT_robotName, '/head/state:o']  signalSize=6  blocking=off  timestamp=off  autoconnect=on  errorOnConnection=off
  Selector1 : Selector  InputPortWidth=6  IndexOptions=Index vector (dialog)  Indices=[1:3]  OutputSizes=1
  Switch : Switch  Criteria=u2 > Threshold
  USE_IMU4EST_BASE1 : Constant  Value=CONFIG.CORRECT_NECK_IMU
  Neck Position : Outport
  wires:
  Head state/1 -> Gain/1
  Selector1/1 -> Switch/1  "neck"
  USE_IMU4EST_BASE1/1 -> Switch/2
  Switch/1 -> Neck Position/1
  Gain/1 -> Selector1/1
  Constant/1 -> Switch/3

== system torqueBalancingR2015a/State Machine/State machine walking/State Machine Walking/visualise inertial/l_sole_H_root_link1/Visualize hom transf7 ==
  H : Inport
  "CoM6D ->  CoMXYZ1" : Selector  NumberOfDimensions=2  InputPortWidth=7  IndexOptions=Index vector (dialog),Index vector (dialog)  Indices=[1 2 3],[1 2 3]  OutputSizes=1,1
  "CoM6D ->  CoMXYZ2" : Selector  NumberOfDimensions=2  InputPortWidth=7  IndexOptions=Index vector (dialog),Index vector (dialog)  Indices=[1 2 3],[4]  OutputSizes=1,1
  Hom : Scope
      settings: TimeRange=auto  LimitDataPoints=on  MaxDataPoints=5000  SaveToWorkspace=off  SaveName=ScopeData  YMin=-10  YMax=10  SampleTime=-1  DataFormat=Array
  R : Scope
      settings: TimeRange=auto  LimitDataPoints=on  MaxDataPoints=5000  SaveToWorkspace=off  SaveName=ScopeData  YMin=-10  YMax=10  SampleTime=-1  DataFormat=Array
  p : Scope
      settings: TimeRange=auto  LimitDataPoints=on  MaxDataPoints=5000  SaveToWorkspace=off  SaveName=ScopeData  YMin=-10  YMax=10  SampleTime=-1  DataFormat=Array
  wires:
  "CoM6D ->  CoMXYZ1"/1 -> R/1
  "CoM6D ->  CoMXYZ2"/1 -> p/1
  H/1 -> "CoM6D ->  CoMXYZ2"/1, Hom/1, "CoM6D ->  CoMXYZ1"/1

== system torqueBalancingR2015a/State Machine/State machine walking/State Machine Walking/visualise inertial/l_sole_H_root_link2/Visualize hom transf7 ==
  H : Inport
  "CoM6D ->  CoMXYZ1" : Selector  NumberOfDimensions=2  InputPortWidth=7  IndexOptions=Index vector (dialog),Index vector (dialog)  Indices=[1 2 3],[1 2 3]  OutputSizes=1,1
  "CoM6D ->  CoMXYZ2" : Selector  NumberOfDimensions=2  InputPortWidth=7  IndexOptions=Index vector (dialog),Index vector (dialog)  Indices=[1 2 3],[4]  OutputSizes=1,1
  Hom : Scope
      settings: TimeRange=auto  LimitDataPoints=on  MaxDataPoints=5000  SaveToWorkspace=off  SaveName=ScopeData  YMin=-10  YMax=10  SampleTime=-1  DataFormat=Array
  R : Scope
      settings: TimeRange=auto  LimitDataPoints=on  MaxDataPoints=5000  SaveToWorkspace=off  SaveName=ScopeData  YMin=-10  YMax=10  SampleTime=-1  DataFormat=Array
  p : Scope
      settings: TimeRange=auto  LimitDataPoints=on  MaxDataPoints=5000  SaveToWorkspace=off  SaveName=ScopeData  YMin=-10  YMax=10  SampleTime=-1  DataFormat=Array
  wires:
  "CoM6D ->  CoMXYZ1"/1 -> R/1
  "CoM6D ->  CoMXYZ2"/1 -> p/1
  H/1 -> "CoM6D ->  CoMXYZ2"/1, Hom/1, "CoM6D ->  CoMXYZ1"/1

== system torqueBalancingR2015a/State Machine/State machine walking/State Machine Walking/visualise inertial/w_H_root_link1/Subsystem ==
  Constant : Constant  Value=zeros(3,1)
  Gain : Gain  Gain=pi/180
  Head state : WBToolboxLibrary/Utilities/Yarp Read  portName=['/',WBT_robotName, '/head/state:o']  signalSize=6  blocking=off  timestamp=off  autoconnect=on  errorOnConnection=off
  Selector1 : Selector  InputPortWidth=6  IndexOptions=Index vector (dialog)  Indices=[1:3]  OutputSizes=1
  Switch : Switch  Criteria=u2 > Threshold
  USE_IMU4EST_BASE1 : Constant  Value=CONFIG.CORRECT_NECK_IMU
  Neck Position : Outport
  wires:
  Head state/1 -> Gain/1
  Selector1/1 -> Switch/1  "neck"
  USE_IMU4EST_BASE1/1 -> Switch/2
  Switch/1 -> Neck Position/1
  Gain/1 -> Selector1/1
  Constant/1 -> Switch/3

== system torqueBalancingR2015a/State Machine/State machine walking/State Machine Walking/visualise inertial/w_H_root_link2/Subsystem ==
  Constant : Constant  Value=zeros(3,1)
  Gain : Gain  Gain=pi/180
  Head state : WBToolboxLibrary/Utilities/Yarp Read  portName=['/',WBT_robotName, '/head/state:o']  signalSize=6  blocking=off  timestamp=off  autoconnect=on  errorOnConnection=off
  Selector1 : Selector  InputPortWidth=6  IndexOptions=Index vector (dialog)  Indices=[1:3]  OutputSizes=1
  Switch : Switch  Criteria=u2 > Threshold
  USE_IMU4EST_BASE1 : Constant  Value=CONFIG.CORRECT_NECK_IMU
  Neck Position : Outport
  wires:
  Head state/1 -> Gain/1
  Selector1/1 -> Switch/1  "neck"
  USE_IMU4EST_BASE1/1 -> Switch/2
  Switch/1 -> Neck Position/1
  Gain/1 -> Selector1/1
  Constant/1 -> Switch/3

== matlab function State Machine/State machine Yoga and Coordinator/State Machine Yoga/visualise inertial/w_H_root_link2/fromImuToHomogeousTransformFCN ==
  data: imu_H_link input double; imu_H_link_0 input double; link_H_root input double; inertial_0 input double; inertial input double; neck input double; w_H_root output double; CONFIG parameter double
function w_H_root = fromBaseToWorldWithImuFCN(imu_H_link,imu_H_link_0,link_H_root,inertial_0,inertial,neck,CONFIG)

    w_H_root = fromBaseToWorldWithImu(imu_H_link,imu_H_link_0,link_H_root,inertial_0,inertial,neck,CONFIG);
end

== matlab function State Machine/State machine Yoga and Coordinator/Internal coordinator/w_H_root_link2/fromImuToHomogeousTransformFCN ==
  data: imu_H_link input double; imu_H_link_0 input double; link_H_root input double; inertial_0 input double; inertial input double; neck input double; w_H_root output double; CONFIG parameter double
function w_H_root = fromBaseToWorldWithImuFCN(imu_H_link,imu_H_link_0,link_H_root,inertial_0,inertial,neck,CONFIG)

    w_H_root = fromBaseToWorldWithImu(imu_H_link,imu_H_link_0,link_H_root,inertial_0,inertial,neck,CONFIG);
end

== matlab function State Machine/State machine Yoga and Coordinator/State Machine Yoga/w_H_root_link1/fromImuToHomogeousTransformFCN ==
  data: imu_H_link input double; imu_H_link_0 input double; link_H_root input double; inertial_0 input double; inertial input double; neck input double; w_H_root output double; CONFIG parameter double
function w_H_root = fromBaseToWorldWithImuFCN(imu_H_link,imu_H_link_0,link_H_root,inertial_0,inertial,neck,CONFIG)

    w_H_root = fromBaseToWorldWithImu(imu_H_link,imu_H_link_0,link_H_root,inertial_0,inertial,neck,CONFIG);
end

== matlab function State Machine/State machine Yoga and Coordinator/State Machine Yoga/visualise inertial/w_H_root_link1/fromImuToHomogeousTransformFCN ==
  data: imu_H_link input double; imu_H_link_0 input double; link_H_root input double; inertial_0 input double; inertial input double; neck input double; w_H_root output double; CONFIG parameter double
function w_H_root = fromBaseToWorldWithImuFCN(imu_H_link,imu_H_link_0,link_H_root,inertial_0,inertial,neck,CONFIG)

    w_H_root = fromBaseToWorldWithImu(imu_H_link,imu_H_link_0,link_H_root,inertial_0,inertial,neck,CONFIG);
end

== matlab function State Machine/State machine walking/State Machine Walking/nu/MATLAB Function ==
  data: JcLeftFoot input double; JcRightFoot input double; activeFeetConstraints input double; y output double; qD input double; reg parameter double
function y = fcn(JcLeftFoot,JcRightFoot,activeFeetConstraints,qD,reg)

    Jc = [activeFeetConstraints(1)*JcLeftFoot;
          activeFeetConstraints(2)*JcRightFoot];

    pinvJb = pinvDamped(Jc(:,1:6),reg.pinvDampVb);  
    y = -pinvJb*Jc(:,7:end)*qD;
end

== matlab function State Machine/State machine walking/State Machine Walking/stateMachineFCN ==
  data: wrench_rightFoot input double; wrench_leftFoot input double; CoMDes output double; CoM_0 input double; q0 input double; x_CoM input double; qj input double; t input double; sm parameter double; impedances output double; kpCom output double; kdCom output double; gain parameter double; currentState output double; CoMDesInput input double; qjDesInput input double; constraintsInput input double
function [CoMDes, impedances, kpCom, kdCom, currentState] =  stateMachineWalkingFCN(...
          wrench_rightFoot,wrench_leftFoot, CoM_0, q0, x_CoM, qj, t, sm, gain, CoMDesInput,...
                                 qjDesInput, constraintsInput)
 
    [CoMDes, impedances, kpCom, kdCom, currentState] = ...
          stateMachineWalking(wrench_rightFoot, wrench_leftFoot, CoM_0, q0, x_CoM, qj, t, sm, gain,...
                              CoMDesInput, qjDesInput, constraintsInput);
end

== matlab function State Machine/State machine Yoga and Coordinator/Internal coordinator/nu/MATLAB Function ==
  data: JcLeftFoot input double; JcRightFoot input double; activeFeetConstraints input double; y output double; qD input double; reg parameter double
function y = fcn(JcLeftFoot,JcRightFoot,activeFeetConstraints,qD,reg)

    Jc = [activeFeetConstraints(1)*JcLeftFoot;
          activeFeetConstraints(2)*JcRightFoot];

    pinvJb = pinvDamped(Jc(:,1:6),reg.pinvDampVb);  
    y = -pinvJb*Jc(:,7:end)*qD;
end

== matlab function State Machine/State machine walking/State Machine Walking/visualise inertial/w_H_root_link1/fromImuToHomogeousTransformFCN ==
  data: imu_H_link input double; imu_H_link_0 input double; link_H_root input double; inertial_0 input double; inertial input double; neck input double; w_H_root output double; CONFIG parameter double
function w_H_root = fromBaseToWorldWithImuFCN(imu_H_link,imu_H_link_0,link_H_root,inertial_0,inertial,neck,CONFIG)

    w_H_root = fromBaseToWorldWithImu(imu_H_link,imu_H_link_0,link_H_root,inertial_0,inertial,neck,CONFIG);
end

== matlab function State Machine/State machine walking/State Machine Walking/visualise inertial/w_H_root_link2/fromImuToHomogeousTransformFCN ==
  data: imu_H_link input double; imu_H_link_0 input double; link_H_root input double; inertial_0 input double; inertial input double; neck input double; w_H_root output double; CONFIG parameter double
function w_H_root = fromBaseToWorldWithImuFCN(imu_H_link,imu_H_link_0,link_H_root,inertial_0,inertial,neck,CONFIG)

    w_H_root = fromBaseToWorldWithImu(imu_H_link,imu_H_link_0,link_H_root,inertial_0,inertial,neck,CONFIG);
end

== matlab function State Machine/State machine Yoga and Coordinator/Internal coordinator/refGen/refGenFCN ==
  data: xCom0 input double; qDes output double; q0 input double; t input double; references parameter double; desired_x_dx_ddx_CoM output double
function [qDes,desired_x_dx_ddx_CoM] = refGenFCN(xCom0,q0,t,references)

    [qDes,desired_x_dx_ddx_CoM] = refGen(xCom0,q0,t,references);
end

== matlab function Controller_QP/integralOf Hw/w_H_root_link2/fromImuToHomogeousTransformFCN ==
  data: imu_H_link input double; imu_H_link_0 input double; link_H_root input double; inertial_0 input double; inertial input double; neck input double; w_H_root output double; CONFIG parameter double
function w_H_root = fromBaseToWorldWithImuFCN(imu_H_link,imu_H_link_0,link_H_root,inertial_0,inertial,neck,CONFIG)

    w_H_root = fromBaseToWorldWithImu(imu_H_link,imu_H_link_0,link_H_root,inertial_0,inertial,neck,CONFIG);
end

== matlab function State Machine/State machine Yoga and Coordinator/State Machine Yoga/nu/MATLAB Function ==
  data: JcLeftFoot input double; JcRightFoot input double; activeFeetConstraints input double; y output double; qD input double; reg parameter double
function y = fcn(JcLeftFoot,JcRightFoot,activeFeetConstraints,qD,reg)

    Jc = [activeFeetConstraints(1)*JcLeftFoot;
          activeFeetConstraints(2)*JcRightFoot];

    pinvJb = pinvDamped(Jc(:,1:6),reg.pinvDampVb);  
    y = -pinvJb*Jc(:,7:end)*qD;
end

== matlab function State Machine/State machine Yoga and Coordinator/State Machine Yoga/stateMachineFCN ==
  data: wrench_rightFoot input double; wrench_leftFoot input double; w_H_b output double; CoMDes output double; qDes output double; constraints output double; CoM_0 input double; q0 input double; l_sole_CoM input double; r_sole_CoM input double; qj input double; t input double; l_sole_H_b input double; r_sole_H_b input double; sm parameter double; impedances output double; kpCom output double; kdCom output double; gain parameter double; currentState output double; jointsSmoothingTime output double
function [w_H_b, CoMDes,qDes,constraints,impedances,kpCom,kdCom,currentState,jointsSmoothingTime] = ...
          stateMachineYogaFCN(wrench_rightFoot, wrench_leftFoot, CoM_0, q0, l_sole_CoM, r_sole_CoM, qj, t, l_sole_H_b, r_sole_H_b, sm, gain)
 
    [w_H_b, CoMDes,qDes,constraints,impedances,kpCom,kdCom,currentState,jointsSmoothingTime] = ...
    stateMachineYoga(CoM_0, q0, l_sole_CoM, r_sole_CoM, qj, t, wrench_rightFoot, wrench_leftFoot, l_sole_H_b, r_sole_H_b, sm, gain); 
end

== matlab function Controller_QP/integralOf Hw/w_H_root_link1/fromImuToHomogeousTransformFCN ==
  data: imu_H_link input double; imu_H_link_0 input double; link_H_root input double; inertial_0 input double; inertial input double; neck input double; w_H_root output double; CONFIG parameter double
function w_H_root = fromBaseToWorldWithImuFCN(imu_H_link,imu_H_link_0,link_H_root,inertial_0,inertial,neck,CONFIG)

    w_H_root = fromBaseToWorldWithImu(imu_H_link,imu_H_link_0,link_H_root,inertial_0,inertial,neck,CONFIG);
end

== matlab function State Machine/State machine walking/State Machine Walking/Compute w_H_b transform/w_H_root_link1/fromImuToHomogeousTransformFCN ==
  data: imu_H_link input double; imu_H_link_0 input double; link_H_root input double; inertial_0 input double; inertial input double; neck input double; w_H_root output double; CONFIG parameter double
function w_H_root = fromBaseToWorldWithImuFCN(imu_H_link,imu_H_link_0,link_H_root,inertial_0,inertial,neck,CONFIG)

    w_H_root = fromBaseToWorldWithImu(imu_H_link,imu_H_link_0,link_H_root,inertial_0,inertial,neck,CONFIG);
end

== matlab function Dump and visualize/plotNorms/norm1 ==
  data: u input double; normU output double
function normU = fcn(u)

    normU = norm(u);
end

== matlab function Controller_QP/tau(f)  ==
  data: tauModel output double; Sigma output double; NA output double; fHdotDesC1C2 output double; HessianMatrixQP1Foot output double; gradientQP1Foot output double; ConstraintsMatrixQP1Foot output double; bVectorConstraintsQp1Foot output double; HessianMatrixQP2Feet output double; gradientQP2Feet output double; ConstraintsMatrixQP2Feet output double; bVectorConstraintsQp2Feet output double; constraints input double; ROBOT_DOF_FOR_SIMULINK input double; ConstraintsMatrix input double; bVectorConstraints input double; q input double; qDes input double; v input double; M input double; h input double; H input double; intHw input double; w_H_l_sole input double; w_H_r_sole input double; JL input double; JR input double; dJLv input double; dJRv input double; xcom input double; J_CoM input double; desired_x_dx_ddx_CoM input double; gainsPCOM input double; gainsDCOM input double; impedances input double; intErrorCoM input double; ki_int_qtilde input double; reg parameter double; gain parameter double; errorCoM output double; qTilde output double; f output double
function [tauModel,Sigma,NA,fHdotDesC1C2, ...
          HessianMatrixQP1Foot,gradientQP1Foot,ConstraintsMatrixQP1Foot,bVectorConstraintsQp1Foot,...
          HessianMatrixQP2Feet,gradientQP2Feet,ConstraintsMatrixQP2Feet,bVectorConstraintsQp2Feet,...
          errorCoM,qTilde,f]    =  ...
          balancingControllerFCN(constraints,ROBOT_DOF_FOR_SIMULINK,ConstraintsMatrix,bVectorConstraints,...
          q,qDes,v, M, h , H,intHw,w_H_l_sole, w_H_r_sole, JL,JR, dJLv,dJRv, xcom,J_CoM, desired_x_dx_ddx_CoM,...
          gainsPCOM,gainsDCOM,impedances, intErrorCoM,ki_int_qtilde,reg,gain)

    % BALANCING CONTROLLER
    [tauModel,Sigma,NA,fHdotDesC1C2, ...
                  HessianMatrixQP1Foot,gradientQP1Foot,ConstraintsMatrixQP1Foot,bVectorConstraintsQp1Foot,...
                  HessianMatrixQP2Feet,gradientQP2Feet,ConstraintsMatrixQP2Feet,bVectorConstraintsQp2Feet,...
                  errorCoM,qTilde,f]    =  ...
                  balancingController(constraints,ROBOT_DOF_FOR_SIMULINK,ConstraintsMatrix,bVectorConstraints,...
                  q,qDes,v, M, h , H,intHw,w_H_l_sole, w_H_r_sole, JL,JR, dJLv,dJRv, xcom,J_CoM, desired_x_dx_ddx_CoM,...
                  gainsPCOM,gainsDCOM,impedances,intErrorCoM,ki_int_qtilde,reg,gain);
end

== matlab function emergency stop: joint limits/MATLAB Function ==
  data: umin input double; umax input double; u input double; inRange output double; tol input double
function inRange = checkRange(umin, umax, u, tol)

    res = u < umin + tol | u > umax - tol;
    res = sum(res);
    if res==0
        inRange = 1;
    else
        inRange = 0;
        u < umin + tol | u > umax - tol;
    end
end
